simulink model "MATLAB_FILE_EV_final"  (R2021a)
settings: Solver=ode45  StartTime=0.0  StopTime=0.5  MaxStep=0.0001  RelTol=1e-3
undefined symbols (not defined in the file): Ion, Lithium
libraries: spsSeriesRLCBranchLib x14, spsIdealSwitchLib x10, pid_lib x9, spsMosfetLib x8, spsPWMGeneratorDCDCLib x6, spsVoltageMeasurementLib x5, spsThreePhaseSeriesRLCLoadLib x4, spsThreePhaseVIMeasurementLib x3, spsThreePhaseBreakerLib x2, spsUniversalBridgeLib x2, spsBatteryLib x1, spsThreePhaseSourceLib x1
(part 1 of 2)
settings Model: Creator=DarkDoom  LastModifiedBy=DarkDoom
settings SolverCC: ZeroCrossControl=DisableAll  SolverResetMethod=Robust

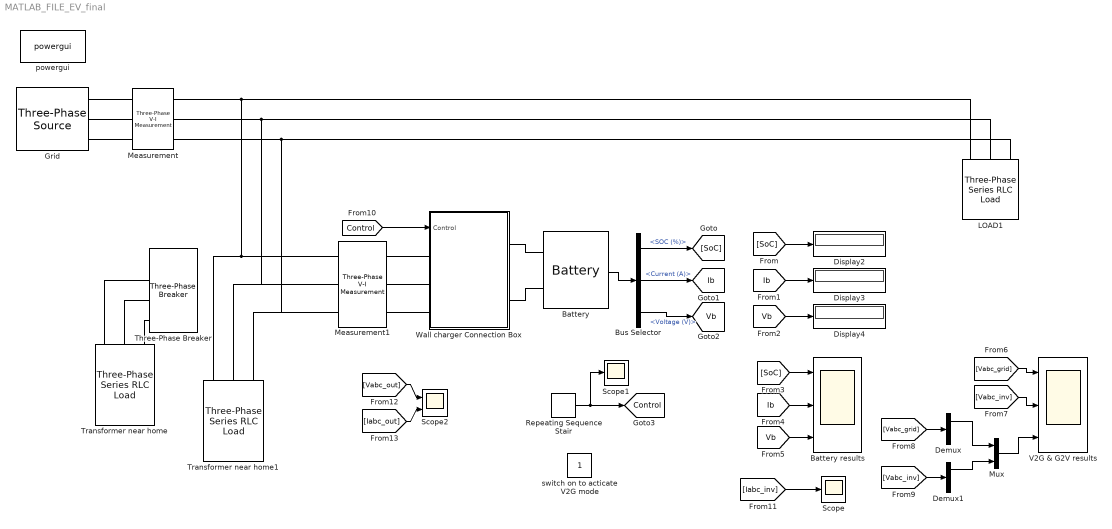
== system MATLAB_FILE_EV_final ==
  Battery : spsBatteryLib/Battery  BatType=Lithium-Ion  ShowTempParam=off  ThermalPreset=no  ShowAgeParam=off  NomV=230  NomQ=100  SOC=60  Batt_Tr=1e-3  PresetModel=on  MaxQ=100  MinV=172.5  FullV=267.717  Dis_rate=43.4783  R=0.023  Normal_OP=90.4348  expZone="[248.4887      4.913043]"  current=[6.5 13 32.5]  Units=Time  Tci=20  NomT=20  T2=-30  MaxQ2=4.8  FullV2=7.1  Normal_OP2=5.655  expZone2="[6.58           1]"  Rca=0.6  ti=2000  Dp=0  Neq0=0  Tsim=1e6  Ta1=25  Qeol=5.4*0.9  Reol=0.013333*1.2  Char_age=[2.3478, 3]  Dis_age=[2.3478, 10]  N1=1500  N2=10500  N3=1000  N4=1400  Ta2=45  N5=950
  Battery results : Scope  NumInputPorts=3
  Bus Selector : BusSelector  OutputSignals=SOC (%),Current (A),Voltage (V)
  Demux : Demux  Outputs=3
  Demux1 : Demux  Outputs=3
  Display2 : Display
  Display3 : Display
  Display4 : Display
  Grid : spsThreePhaseSourceLib/Three-Phase Source  InternalConnection=Yg  VoltagePhases=off  Voltage=380  PhaseAngle=0  Voltage_phases=[25e3 25e3 25e3]/sqrt(3)  PhaseAngles_phases=[0 -120 +120]  Frequency=50  NonIdealSource=on  SpecifyImpedance=on  Resistance=0.8929  Inductance=16.58e-3  ShortCircuitLevel=100e6  BaseVoltage=380  XRratio=7  BusType=swing  Pref=10e3  Qref=0  Prefabc=[10e3, 10e3, 10e3]  Qrefabc=[0, 0, 0]  Qmin=-inf  Qmax=inf
  LOAD1 : spsThreePhaseSeriesRLCLoadLib/Three-Phase Series RLC Load  LConnTagsString=A|B|C  Configuration=Y (grounded)  NominalVoltage=380  Vabc=[1e3 1e3 1e3]  Vabcp=[1e3 1e3 1e3]  NominalFrequency=50  UnbalancedPower=off  ActivePower=1e3  InductivePower=0  CapacitivePower=0  Pabc=[10e3 9e3 11e3]  QLabc=[100 90 110]  QCabc=[100 90 110]  Pabcp=[10e3 9e3 11e3]  QLabcp=[100 90 110]  QCabcp=[100 90 110]  Measurements=None  LoadType=constant Z
  Measurement : spsThreePhaseVIMeasurementLib/Three-Phase V-I Measurement  VoltageMeasurement=phase-to-ground  SetLabelV=on  LabelV=Vabc_grid  Vpu=off  VpuLL=off  CurrentMeasurement=yes  SetLabelI=on  LabelI=Iabc_grid  Ipu=off  Pbase=100e6  Vbase=500e3  OutputType=Complex  PhasorSimulation=off  PSBequivalent=0
  Measurement1 : spsThreePhaseVIMeasurementLib/Three-Phase V-I Measurement  VoltageMeasurement=phase-to-ground  SetLabelV=on  LabelV=Vabc_out  Vpu=off  VpuLL=off  CurrentMeasurement=yes  SetLabelI=on  LabelI=Iabc_out  Ipu=off  Pbase=100e6  Vbase=500e3  OutputType=Complex  PhasorSimulation=off  PSBequivalent=0
  Mux : Mux  Inputs=2
  Repeating Sequence Stair : simulink/Sources/Repeating Sequence Stair  OutValues=[0 0 1 1 0].'  tsamp=0.1  OutMin=[]  OutMax=[]  OutDataTypeStr=double  OutputDataTypeScalingMode=double  OutDataType=fixdt(0,8)  ConRadixGroup=Best Precision: Vector-wise  OutScaling=2^-12
  Scope : Scope
  Scope1 : Scope
  Scope2 : Scope  NumInputPorts=2
  Three-Phase Breaker : spsThreePhaseBreakerLib/Three-Phase Breaker  InitialState=open  SwitchA=on  SwitchB=on  SwitchC=on  SwitchTimes="[0.1  0.25]"  External=on  BreakerResistance=0.01  SnubberResistance=1e6  SnubberCapacitance=inf  Measurements=None
  Transformer near home : spsThreePhaseSeriesRLCLoadLib/Three-Phase Series RLC Load  LConnTagsString=A|B|C  Configuration=Y (grounded)  NominalVoltage=380  Vabc=[1e3 1e3 1e3]  Vabcp=[1e3 1e3 1e3]  NominalFrequency=50  UnbalancedPower=off  ActivePower=20e3  InductivePower=0  CapacitivePower=0  Pabc=[10e3 9e3 11e3]  QLabc=[100 90 110]  QCabc=[100 90 110]  Pabcp=[10e3 9e3 11e3]  QLabcp=[100 90 110]  QCabcp=[100 90 110]  Measurements=None  LoadType=constant Z
  Transformer near home1 : spsThreePhaseSeriesRLCLoadLib/Three-Phase Series RLC Load  LConnTagsString=A|B|C  Configuration=Y (grounded)  NominalVoltage=380  Vabc=[1e3 1e3 1e3]  Vabcp=[1e3 1e3 1e3]  NominalFrequency=50  UnbalancedPower=off  ActivePower=1e3  InductivePower=0  CapacitivePower=0  Pabc=[10e3 9e3 11e3]  QLabc=[100 90 110]  QCabc=[100 90 110]  Pabcp=[10e3 9e3 11e3]  QLabcp=[100 90 110]  QCabcp=[100 90 110]  Measurements=None  LoadType=constant Z
  V2G & G2V results : Scope  NumInputPorts=3
  Wall charger Connection Box : Subsystem
  powergui : spspowerguiLib/powergui  Priority=1  SimulationMode=Discrete  SampleTime=50e-6  frequency=60  Iterations=50  frequencyindice=0  Pbase=100e6  ErrMax=1e-4  UnitsV=kV  UnitsW=MW  buscounter=0  FunctionMessages=off  echomessages=off  EnableUseOfTLC=off  CurrentSourceSwitches=off  DisableSnubberDevices=off  DisableRonSwitches=off  DisableVfSwitches=off  DisplayEquations=off  AutomaticDiscreteSolvers=off  SolverType=Tustin/Backward Euler (TBE)  Interpol=off  ExternalGateDelay=off  methode=off  Ts=100  x0status=blocks  SPID=on  SwTol=0  HookPort=off  NonlinearTolerance=1e-4  nMaxIteration=100  ContinueOnMaxIteration=off  RestoreLinks=warning  ResistiveCurrentMeasurement=off  Frange=[0:2:500]  Ylog=off  Xlog=on  ShowGrid=off  save=off  variable=ZData  structure=0  ZoomFFT=off  StartTime=0.0  cycles=1  DisplayStyle=1  fundamental=60  FreqAxis=off  MaxFrequency=1000  frequencyindicesteady=1  RmsSteady=1  display=off
  switch on to acticate V2G mode : Constant  VectorParams1D=off
  tag scope: Control=global, Ib=global, Vb=global
  wires:
  [Control] -> Wall charger Connection Box/1(Control)
  Battery/1 -> Bus Selector/1
  Bus Selector/1 -> [SoC]  "<SOC (%)>"
  Bus Selector/2 -> [Ib]  "<Current (A)>"
  Bus Selector/3 -> [Vb]  "<Voltage (V)>"
  [SoC] -> Display2/1
  [Ib] -> Display3/1
  [Vb] -> Display4/1
  [SoC] -> Battery results/1
  [Ib] -> Battery results/2
  [Vb] -> Battery results/3
  [Vabc_grid] -> V2G & G2V results/1
  [Vabc_inv] -> V2G & G2V results/2
  [Vabc_grid] -> Demux/1
  [Vabc_inv] -> Demux1/1
  Demux/1 -> Mux/1
  Demux1/1 -> Mux/2
  Mux/1 -> V2G & G2V results/3
  [Iabc_inv] -> Scope/1
  Repeating Sequence Stair/1 -> [Control], Scope1/1
  [Vabc_out] -> Scope2/1
  [Iabc_out] -> Scope2/2
  connections:
  Grid/RConn1 -- Measurement/LConn1
  Grid/RConn2 -- Measurement/LConn2
  Grid/RConn3 -- Measurement/LConn3
  Transformer near home/LConn1 -- Three-Phase Breaker/LConn1
  Transformer near home/LConn2 -- Three-Phase Breaker/LConn2
  Transformer near home1/LConn3 -- Measurement1/LConn3 -- LOAD1/LConn3 -- Measurement/RConn3
  Wall charger Connection Box/RConn1 -- Battery/LConn1
  Wall charger Connection Box/RConn2 -- Battery/LConn2
  Wall charger Connection Box/LConn2 -- Measurement1/RConn2
  Wall charger Connection Box/LConn1 -- Measurement1/RConn1
  Wall charger Connection Box/LConn3 -- Measurement1/RConn3
  Transformer near home/LConn3 -- Three-Phase Breaker/LConn3
  Measurement1/LConn1 -- Transformer near home1/LConn1 -- Measurement/RConn1 -- LOAD1/LConn1
  Measurement/RConn2 -- Transformer near home1/LConn2 -- Measurement1/LConn2 -- LOAD1/LConn2

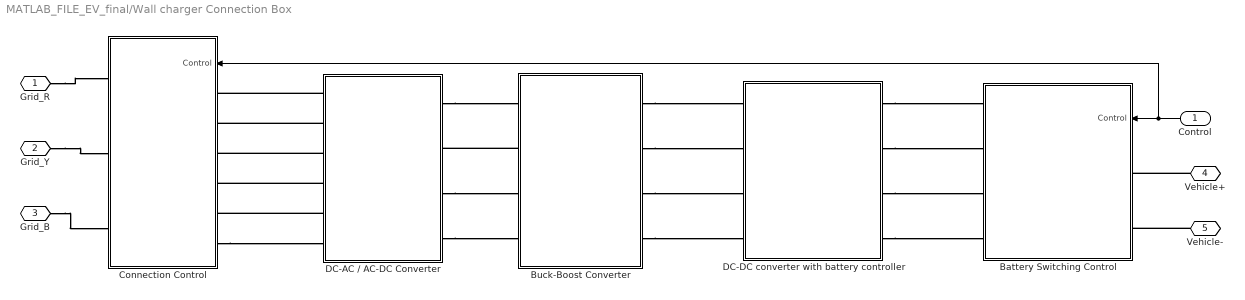
== system MATLAB_FILE_EV_final/Wall charger Connection Box ==
  Control : Inport
  Battery Switching Control : Subsystem
      settings: PortSchema="{\"entries\":[{\"content\":{\"sides\":[{\"content\":{\"connectorIds\":[\"LConn1\",\"LConn2\",\"LConn3\",\"LConn4\"]},\"type\":\"ConnectorPlacement.EquallySpacedRectSide\",\"uuid\":\"597ce45f-d2da-489f-9702-c83ae9b1152a\"},{\"content\":{\"connectorIds\":[\"In1\",\"RConn1\",\"RConn2\"],\"side\":\"RIGHT\"},\"type\":\"ConnectorPlacement.EquallySpacedRectSide\",\"uuid\":\"90ab1945-2787-45d6-b647-1c8eb49fe34d\"},{\"content\":{\"connectorIds\":[],\"side\":\"TOP\"},\"type\":\"ConnectorPlacement.EquallySpacedRectSide\",\"uuid\":\"5514c8fd-a1bb-4ed7-b1c0-08bce6a0e9e5\"}]},\"type\":\"ConnectorPlacement.EquallySpacedConnector\",\"uuid\":\"b6d566cb-31ba-40ab-ae9a-003997b713cb\"}],\"packageUris\":[\"http://schema.mathworks.com/mf0/Connector/R2020b\"],\"version\":\"1.0\"}"
  Buck-Boost Converter : Subsystem
  Connection Control : Subsystem
      settings: PortSchema="{\"entries\":[{\"content\":{\"sides\":[{\"content\":{\"connectorIds\":[\"LConn1\",\"LConn2\",\"LConn3\"]},\"type\":\"ConnectorPlacement.EquallySpacedRectSide\",\"uuid\":\"27ebf5cb-61b2-431e-8de2-c9344a0dfca5\"},{\"content\":{\"connectorIds\":[\"In1\",\"RConn1\",\"RConn2\",\"RConn3\",\"RConn4\",\"RConn5\",\"RConn6\"],\"side\":\"RIGHT\"},\"type\":\"ConnectorPlacement.EquallySpacedRectSide\",\"uuid\":\"2438100a-e43b-42f7-afa1-1af449516139\"},{\"content\":{\"connectorIds\":[],\"side\":\"TOP\"},\"type\":\"ConnectorPlacement.EquallySpacedRectSide\",\"uuid\":\"dcfa608d-f6dc-42e3-abf8-45a08af22825\"}]},\"type\":\"ConnectorPlacement.EquallySpacedConnector\",\"uuid\":\"5f0f36e8-f735-4489-a6f2-39fec655b509\"}],\"packageUris\":[\"http://schema.mathworks.com/mf0/Connector/R2020b\"],\"version\":\"1.0\"}"
  DC-AC / AC-DC Converter : Subsystem
  DC-DC converter with battery controller : Subsystem
  Grid_R : PMIOPort  Side=Left
  Grid_Y : PMIOPort  Port=2  Side=Left
  Grid_B : PMIOPort  Port=3  Side=Left
  Vehicle+ : PMIOPort  Port=4  Side=Right
  Vehicle- : PMIOPort  Port=5  Side=Right
  wires:
  Control/1 -> Connection Control/1(Control), Battery Switching Control/1(Control)
  connections:
  DC-AC / AC-DC Converter/LConn5 -- Connection Control/RConn5
  DC-AC / AC-DC Converter/LConn2 -- Connection Control/RConn2
  DC-DC converter with battery controller/RConn3 -- Battery Switching Control/LConn3
  Buck-Boost Converter/RConn2 -- DC-DC converter with battery controller/LConn2
  Grid_B/RConn1 -- Connection Control/LConn3
  DC-AC / AC-DC Converter/RConn3 -- Buck-Boost Converter/LConn3
  Grid_R/RConn1 -- Connection Control/LConn1
  DC-AC / AC-DC Converter/LConn1 -- Connection Control/RConn1
  Vehicle-/RConn1 -- Battery Switching Control/RConn2
  Vehicle+/RConn1 -- Battery Switching Control/RConn1
  Buck-Boost Converter/RConn4 -- DC-DC converter with battery controller/LConn4
  Grid_Y/RConn1 -- Connection Control/LConn2
  DC-AC / AC-DC Converter/LConn4 -- Connection Control/RConn4
  DC-DC converter with battery controller/RConn2 -- Battery Switching Control/LConn2
  DC-DC converter with battery controller/RConn1 -- Battery Switching Control/LConn1
  DC-DC converter with battery controller/RConn4 -- Battery Switching Control/LConn4
  Buck-Boost Converter/RConn1 -- DC-DC converter with battery controller/LConn1
  Buck-Boost Converter/LConn2 -- DC-AC / AC-DC Converter/RConn2
  DC-AC / AC-DC Converter/LConn3 -- Connection Control/RConn3
  DC-AC / AC-DC Converter/RConn1 -- Buck-Boost Converter/LConn1
  DC-AC / AC-DC Converter/RConn4 -- Buck-Boost Converter/LConn4
  Buck-Boost Converter/RConn3 -- DC-DC converter with battery controller/LConn3
  Connection Control/RConn6 -- DC-AC / AC-DC Converter/LConn6

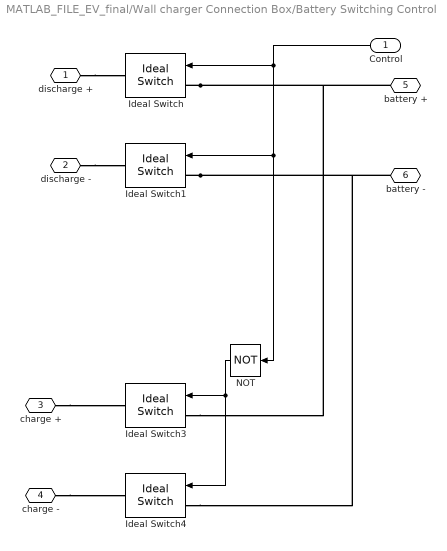
== system MATLAB_FILE_EV_final/Wall charger Connection Box/Battery Switching Control ==
  Control : Inport
  Ideal Switch{,1,3..4} (4 alike) : spsIdealSwitchLib/Ideal Switch  Ron=0.001  Lon=0  IC=0  Rs=1e5  Cs=inf  Measurements=off
  NOT : Logic  Operator=NOT  IconShape=distinctive  AllPortsSameDT=off  OutDataTypeStr=boolean
  discharge + : PMIOPort  Side=Left
  discharge - : PMIOPort  Port=2  Side=Left
  charge + : PMIOPort  Port=3  Side=Left
  charge - : PMIOPort  Port=4  Side=Left
  battery + : PMIOPort  Port=5  Side=Right
  battery - : PMIOPort  Port=6  Side=Right
  wires:
  Control/1 -> NOT/1, Ideal Switch1/1, Ideal Switch/1
  NOT/1 -> Ideal Switch4/1, Ideal Switch3/1
  connections:
  charge -/RConn1 -- Ideal Switch4/RConn1
  discharge +/RConn1 -- Ideal Switch/RConn1
  Ideal Switch1/LConn1 -- battery -/RConn1 -- Ideal Switch4/LConn1
  discharge -/RConn1 -- Ideal Switch1/RConn1
  Ideal Switch/LConn1 -- battery +/RConn1 -- Ideal Switch3/LConn1
  charge +/RConn1 -- Ideal Switch3/RConn1

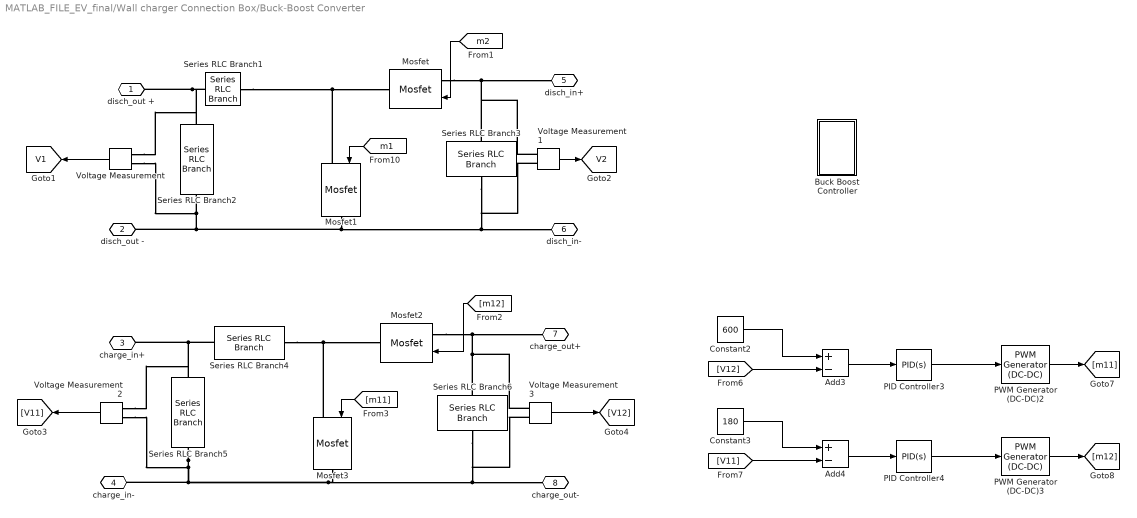
== system MATLAB_FILE_EV_final/Wall charger Connection Box/Buck-Boost Converter ==
  Add3 : Sum  Inputs=+-
  Add4 : Sum  Inputs=+-
  Buck Boost Controller : Subsystem
  Constant2 : Constant  Value=600
  Constant3 : Constant  Value=180
  Mosfet{,1..3} (4 alike) : spsMosfetLib/Mosfet  Ron=0.1  Lon=0  Rd=0.01  Vfd=0  IC=0  Rs=1e5  Cs=inf  Measurements=off
  PID Controller3 : pid_lib/PID Controller  Controller=PID  Form=Parallel  TimeDomain=Continuous-time  UseExternalTs=off  SampleTime=-1  IntegratorMethod=Forward Euler  FilterMethod=Forward Euler  ControllerParametersSource=internal  P=0  I=7  D=0  UseFilter=on  N=100  TunerSelectOption=Transfer Function Based (PID Tuner App)  InitialConditionSource=internal  InitialConditionForIntegrator=0  InitialConditionForFilter=0  DifferentiatorICPrevScaledInput=0  ExternalReset=none  TrackingMode=off  Kt=1  LimitOutput=off  SatLimitsSource=internal  UpperSaturationLimit=inf  LowerSaturationLimit=-inf  LinearizeAsGain=on  AntiWindupMode=none  Kb=1  POutMin=[]  POutMax=[]  IOutMin=[]  IOutMax=[]  DOutMin=[]  DOutMax=[]  NOutMin=[]  NOutMax=[]  SumOutMin=[]  SumOutMax=[]  SaturationOutMin=[]  SaturationOutMax=[]  PParamMin=[]  PParamMax=[]  IParamMin=[]  IParamMax=[]  DParamMin=[]  DParamMax=[]  NParamMin=[]  NParamMax=[]  KbParamMin=[]  KbParamMax=[]  KtParamMin=[]  KtParamMax=[]  KbOutMin=[]  KbOutMax=[]  KtOutMin=[]  KtOutMax=[]  IntegratorOutMin=[]  IntegratorOutMax=[]  FilterOutMin=[]  FilterOutMax=[]  SumI1OutMin=[]  SumI1OutMax=[]  SumI2OutMin=[]  SumI2OutMax=[]  SumI3OutMin=[]  SumI3OutMax=[]  SumI4OutMin=[]  SumI4OutMax=[]  SumDOutMin=[]  SumDOutMax=[]  DifferentiatorOutMin=[]  DifferentiatorOutMax=[]  FilterDiffOutCoefMin=[]  FilterDiffOutCoefMax=[]  ReciprocalOutMin=[]  ReciprocalOutMax=[]  SumDenOutMin=[]  SumDenOutMax=[]  SumNumOutMin=[]  SumNumOutMax=[]  DivideOutMin=[]  DivideOutMax=[]  UdiffTsProdOutMin=[]  UdiffTsProdOutMax=[]  NTsProdOutMin=[]  NTsProdOutMax=[]  UintegralTsProdOutMin=[]  UintegralTsProdOutMax=[]  UngainTsProdOutMin=[]  UngainTsProdOutMax=[]  IntegratorContinuousStateAttributes=''  IntegratorStateMustResolveToSignalObject=off  IntegratorRTWStateStorageClass=Auto  FilterContinuousStateAttributes=''  FilterStateMustResolveToSignalObject=off  FilterRTWStateStorageClass=Auto  ParallelPVariant=InternalParameters  IdealPVariant=Disabled  IVariant=InternalParameters  DVariant=InternalParameters  IntegratorVariant=Continuous  SatVariant=Disabled  AWVariant=Passthrough  PCopyVariant=Disabled  TRVariant=Disabled  FdbkBlocksVariant=Forward  IdealPFdbkVariant=Disabled  SatFdbkVariant=Disabled  DerivativeFilterVariant=ContFilter  NVariant=InternalParameters  NCopyVariant=Disabled  FilterICVariant=InternalICsFilter  IntegratorICVariant=InternalICs  ExternalResetVariant=Disabled  TRSumVariant=Passthrough  SumFdbkVariant=Disabled  SumVariant=Sum_PID  TsampFilterVariant=InternalTs  TsampNgainVariant=Passthrough  TsampIntegralVariant=Passthrough  ExternalSaturationOutDataTypeStr=Inherit: Same as second input
  PID Controller4 : pid_lib/PID Controller  Controller=PID  Form=Parallel  TimeDomain=Continuous-time  UseExternalTs=off  SampleTime=-1  IntegratorMethod=Forward Euler  FilterMethod=Forward Euler  ControllerParametersSource=internal  P=0  I=7  D=0  UseFilter=on  N=100  TunerSelectOption=Transfer Function Based (PID Tuner App)  InitialConditionSource=internal  InitialConditionForIntegrator=0  InitialConditionForFilter=0  DifferentiatorICPrevScaledInput=0  ExternalReset=none  TrackingMode=off  Kt=1  LimitOutput=off  SatLimitsSource=internal  UpperSaturationLimit=inf  LowerSaturationLimit=-inf  LinearizeAsGain=on  AntiWindupMode=none  Kb=1  POutMin=[]  POutMax=[]  IOutMin=[]  IOutMax=[]  DOutMin=[]  DOutMax=[]  NOutMin=[]  NOutMax=[]  SumOutMin=[]  SumOutMax=[]  SaturationOutMin=[]  SaturationOutMax=[]  PParamMin=[]  PParamMax=[]  IParamMin=[]  IParamMax=[]  DParamMin=[]  DParamMax=[]  NParamMin=[]  NParamMax=[]  KbParamMin=[]  KbParamMax=[]  KtParamMin=[]  KtParamMax=[]  KbOutMin=[]  KbOutMax=[]  KtOutMin=[]  KtOutMax=[]  IntegratorOutMin=[]  IntegratorOutMax=[]  FilterOutMin=[]  FilterOutMax=[]  SumI1OutMin=[]  SumI1OutMax=[]  SumI2OutMin=[]  SumI2OutMax=[]  SumI3OutMin=[]  SumI3OutMax=[]  SumI4OutMin=[]  SumI4OutMax=[]  SumDOutMin=[]  SumDOutMax=[]  DifferentiatorOutMin=[]  DifferentiatorOutMax=[]  FilterDiffOutCoefMin=[]  FilterDiffOutCoefMax=[]  ReciprocalOutMin=[]  ReciprocalOutMax=[]  SumDenOutMin=[]  SumDenOutMax=[]  SumNumOutMin=[]  SumNumOutMax=[]  DivideOutMin=[]  DivideOutMax=[]  UdiffTsProdOutMin=[]  UdiffTsProdOutMax=[]  NTsProdOutMin=[]  NTsProdOutMax=[]  UintegralTsProdOutMin=[]  UintegralTsProdOutMax=[]  UngainTsProdOutMin=[]  UngainTsProdOutMax=[]  IntegratorContinuousStateAttributes=''  IntegratorStateMustResolveToSignalObject=off  IntegratorRTWStateStorageClass=Auto  FilterContinuousStateAttributes=''  FilterStateMustResolveToSignalObject=off  FilterRTWStateStorageClass=Auto  ParallelPVariant=InternalParameters  IdealPVariant=Disabled  IVariant=InternalParameters  DVariant=InternalParameters  IntegratorVariant=Continuous  SatVariant=Disabled  AWVariant=Passthrough  PCopyVariant=Disabled  TRVariant=Disabled  FdbkBlocksVariant=Forward  IdealPFdbkVariant=Disabled  SatFdbkVariant=Disabled  DerivativeFilterVariant=ContFilter  NVariant=InternalParameters  NCopyVariant=Disabled  FilterICVariant=InternalICsFilter  IntegratorICVariant=InternalICs  ExternalResetVariant=Disabled  TRSumVariant=Passthrough  SumFdbkVariant=Disabled  SumVariant=Sum_PID  TsampFilterVariant=InternalTs  TsampNgainVariant=Passthrough  TsampIntegralVariant=Passthrough  ExternalSaturationOutDataTypeStr=Inherit: Same as second input
  PWM Generator (DC-DC)2 : spsPWMGeneratorDCDCLib/PWM Generator (DC-DC)  Fsw=5000  Ts=0
  PWM Generator (DC-DC)3 : spsPWMGeneratorDCDCLib/PWM Generator (DC-DC)  Fsw=5000  Ts=0
  Series RLC Branch1 : spsSeriesRLCBranchLib/Series RLC Branch  LConnTagsString=__new0  RConnTagsString=__new0  BranchType=L  Resistance=1  Inductance=1e-3  SetiL0=off  InitialCurrent=0  Capacitance=1e-6  Setx0=off  InitialVoltage=0  Measurements=None
  Series RLC Branch{2..3,5..6} (4 alike) : spsSeriesRLCBranchLib/Series RLC Branch  LConnTagsString=__new0  RConnTagsString=__new0  BranchType=RC  Resistance=0.0001  Inductance=1e-3  SetiL0=off  InitialCurrent=0  Capacitance=1000e-6  Setx0=off  InitialVoltage=0  Measurements=None
  Series RLC Branch4 : spsSeriesRLCBranchLib/Series RLC Branch  LConnTagsString=__new0  RConnTagsString=__new0  BranchType=L  Resistance=100e3  Inductance=1e-3  SetiL0=off  InitialCurrent=0  Capacitance=1e-6  Setx0=off  InitialVoltage=0  Measurements=None
  Voltage Measurement{,1..3} (4 alike) : spsVoltageMeasurementLib/Voltage Measurement  PhasorSimulation=off  OutputType=Complex  PSBequivalent=0
  disch_out + : PMIOPort  Side=Left
  disch_out - : PMIOPort  Port=2  Side=Left
  charge_in+ : PMIOPort  Port=3  Side=Left
  charge_in- : PMIOPort  Port=4  Side=Left
  disch_in+ : PMIOPort  Port=5  Side=Right
  disch_in- : PMIOPort  Port=6  Side=Right
  charge_out+ : PMIOPort  Port=7  Side=Right
  charge_out- : PMIOPort  Port=8  Side=Right
  tag scope: V1=global, V2=global
  wires:
  Voltage Measurement1/1 -> [V2]
  Voltage Measurement/1 -> [V1]
  PWM Generator (DC-DC)2/1 -> [m11]
  [V11] -> Add4/2
  Add3/1 -> PID Controller3/1
  Voltage Measurement3/1 -> [V12]
  PID Controller4/1 -> PWM Generator (DC-DC)3/1
  PID Controller3/1 -> PWM Generator (DC-DC)2/1
  Add4/1 -> PID Controller4/1
  [m11] -> Mosfet3/1
  Voltage Measurement2/1 -> [V11]
  PWM Generator (DC-DC)3/1 -> [m12]
  [m12] -> Mosfet2/1
  Constant3/1 -> Add4/1
  Constant2/1 -> Add3/1
  [V12] -> Add3/2
  [m1] -> Mosfet1/1
  [m2] -> Mosfet/1
  connections:
  Series RLC Branch5/RConn1 -- charge_in-/RConn1 -- charge_out-/RConn1 -- Voltage Measurement3/LConn2 -- Series RLC Branch6/RConn1 -- Mosfet3/RConn1 -- Voltage Measurement2/LConn2
  Mosfet1/RConn1 -- disch_in-/RConn1 -- Voltage Measurement1/LConn2 -- Series RLC Branch3/RConn1 -- disch_out -/RConn1 -- Voltage Measurement/LConn2 -- Series RLC Branch2/RConn1
  Mosfet/LConn1 -- disch_in+/RConn1 -- Voltage Measurement1/LConn1 -- Series RLC Branch3/LConn1
  Series RLC Branch4/LConn1 -- charge_in+/RConn1 -- Voltage Measurement2/LConn1 -- Series RLC Branch5/LConn1
  Series RLC Branch1/LConn1 -- Voltage Measurement/LConn1 -- Series RLC Branch2/LConn1 -- disch_out +/RConn1
  Series RLC Branch6/LConn1 -- Voltage Measurement3/LConn1 -- charge_out+/RConn1 -- Mosfet2/LConn1
  Mosfet1/LConn1 -- Series RLC Branch1/RConn1 -- Mosfet/RConn1
  Series RLC Branch4/RConn1 -- Mosfet3/LConn1 -- Mosfet2/RConn1

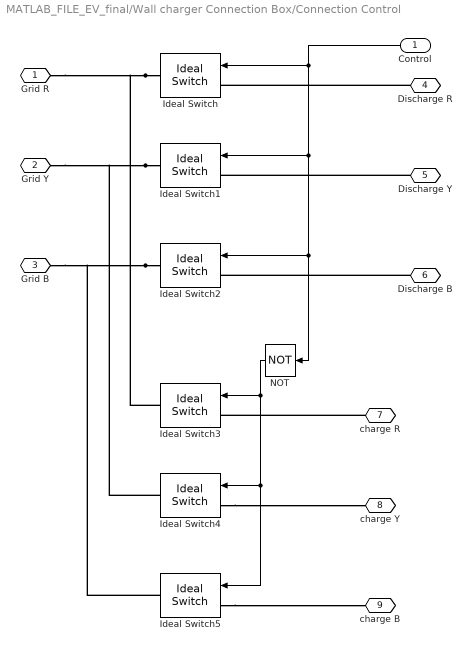
== system MATLAB_FILE_EV_final/Wall charger Connection Box/Connection Control ==
  Control : Inport
  Ideal Switch{,1..5} (6 alike) : spsIdealSwitchLib/Ideal Switch  Ron=0.001  Lon=0  IC=0  Rs=1e5  Cs=inf  Measurements=off
  NOT : Logic  Operator=NOT  IconShape=distinctive  AllPortsSameDT=off  OutDataTypeStr=boolean
  Grid R : PMIOPort  Side=Left
  Grid Y : PMIOPort  Port=2  Side=Left
  Grid B : PMIOPort  Port=3  Side=Left
  Discharge R : PMIOPort  Port=4  Side=Right
  Discharge Y : PMIOPort  Port=5  Side=Right
  Discharge B : PMIOPort  Port=6  Side=Right
  charge R : PMIOPort  Port=7  Side=Right
  charge Y : PMIOPort  Port=8  Side=Right
  charge B : PMIOPort  Port=9  Side=Right
  wires:
  Control/1 -> NOT/1, Ideal Switch2/1, Ideal Switch1/1, Ideal Switch/1
  NOT/1 -> Ideal Switch5/1, Ideal Switch4/1, Ideal Switch3/1
  connections:
  Ideal Switch2/RConn1 -- Grid B/RConn1 -- Ideal Switch5/RConn1
  Discharge R/RConn1 -- Ideal Switch/LConn1
  Discharge B/RConn1 -- Ideal Switch2/LConn1
  Ideal Switch/RConn1 -- Grid R/RConn1 -- Ideal Switch3/RConn1
  Ideal Switch1/RConn1 -- Grid Y/RConn1 -- Ideal Switch4/RConn1
  Ideal Switch4/LConn1 -- charge Y/RConn1
  Discharge Y/RConn1 -- Ideal Switch1/LConn1
  charge R/RConn1 -- Ideal Switch3/LConn1
  Ideal Switch5/LConn1 -- charge B/RConn1

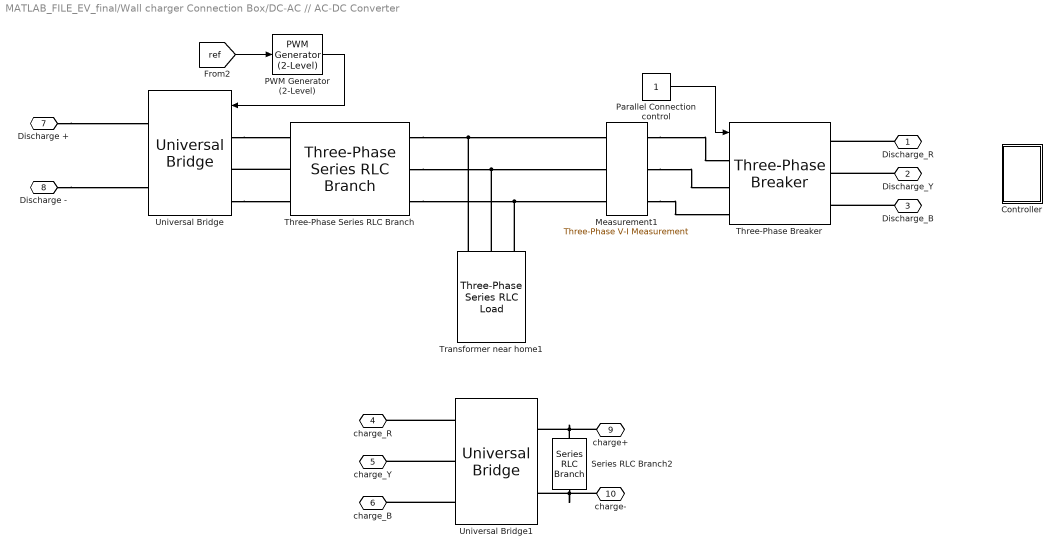
== system MATLAB_FILE_EV_final/Wall charger Connection Box/DC-AC // AC-DC Converter ==
  Controller : Subsystem
  Measurement1 : spsThreePhaseVIMeasurementLib/Three-Phase V-I Measurement  VoltageMeasurement=phase-to-ground  SetLabelV=on  LabelV=Vabc_inv  Vpu=off  VpuLL=off  CurrentMeasurement=yes  SetLabelI=on  LabelI=Iabc_inv  Ipu=off  Pbase=100e6  Vbase=500e3  OutputType=Complex  PhasorSimulation=off  PSBequivalent=0
  PWM Generator (2-Level) : spsPWMGenerator2LevelLib/PWM Generator (2-Level)  ModulatorType=Three-phase bridge (6 pulses)  ModulatorMode=Unsynchronized  Fc=4950  Pc=90  nF=27  MinMax="[ -1  1 ]"  SamplingTechnique=Natural  ModulatingSignals=off  m=0.8  Freq=60  Phase=0  Ts=2.02e-6  ShowCarrierOutport=off
  Parallel Connection control : Constant
  Series RLC Branch2 : spsSeriesRLCBranchLib/Series RLC Branch  LConnTagsString=__new0  RConnTagsString=__new0  BranchType=RC  Resistance=10e3  Inductance=1e-3  SetiL0=off  InitialCurrent=0  Capacitance=1000e-6  Setx0=off  InitialVoltage=0  Measurements=None
  Three-Phase Series RLC Branch : spsThreePhaseSeriesRLCBranchLib/Three-Phase Series RLC Branch  LConnTagsString=A|B|C  RConnTagsString=A|B|C  BranchType=RL  Resistance=0.004332  Inductance=0.0013789184  Capacitance=1e-6  Measurements=None
  Three-Phase Breaker : spsThreePhaseBreakerLib/Three-Phase Breaker  InitialState=open  SwitchA=on  SwitchB=on  SwitchC=on  SwitchTimes="[1/60  5/60]"  External=on  BreakerResistance=0.01  SnubberResistance=1e6  SnubberCapacitance=inf  Measurements=None
  Transformer near home1 : spsThreePhaseSeriesRLCLoadLib/Three-Phase Series RLC Load  LConnTagsString=A|B|C  Configuration=Delta  NominalVoltage=380  Vabc=[1e3 1e3 1e3]  Vabcp=[1e3 1e3 1e3]  NominalFrequency=50  UnbalancedPower=off  ActivePower=100  InductivePower=0  CapacitivePower=5000  Pabc=[10e3 9e3 11e3]  QLabc=[100 90 110]  QCabc=[100 90 110]  Pabcp=[10e3 9e3 11e3]  QLabcp=[100 90 110]  QCabcp=[100 90 110]  Measurements=None  LoadType=constant Z
  Universal Bridge : spsUniversalBridgeLib/Universal Bridge  Arms=3  SnubberResistance=1e5  SnubberCapacitance=inf  Device=IGBT / Diodes  Ron=1e-3  Lon=0  ForwardVoltages="[  0  0  ]"  ForwardVoltage=0  GTOparameters=[ 10e-6 , 20e-6 ]  IGBTparameters=[ 1e-6 , 2e-6 ]  Measurements=None  Measurements_2=None  converterType=Rectifier
  Universal Bridge1 : spsUniversalBridgeLib/Universal Bridge  Arms=3  SnubberResistance=1e5  SnubberCapacitance=inf  Device=Diodes  Ron=1e-3  Lon=0  ForwardVoltages="[  0  0  ]"  ForwardVoltage=0  GTOparameters=[ 10e-6 , 20e-6 ]  IGBTparameters=[ 1e-6 , 2e-6 ]  Measurements=None  Measurements_2=None  converterType=Rectifier
  Discharge_R : PMIOPort  Side=Left
  Discharge_Y : PMIOPort  Port=2  Side=Left
  Discharge_B : PMIOPort  Port=3  Side=Left
  charge_R : PMIOPort  Port=4  Side=Left
  charge_Y : PMIOPort  Port=5  Side=Left
  charge_B : PMIOPort  Port=6  Side=Left
  Discharge + : PMIOPort  Port=7  Side=Right
  Discharge - : PMIOPort  Port=8  Side=Right
  charge+ : PMIOPort  Port=9  Side=Right
  charge- : PMIOPort  Port=10  Side=Right
  wires:
  PWM Generator (2-Level)/1 -> Universal Bridge/1
  Parallel Connection control/1 -> Three-Phase Breaker/1
  [ref] -> PWM Generator (2-Level)/1
  connections:
  Universal Bridge1/LConn2 -- charge_Y/RConn1
  Universal Bridge1/LConn3 -- charge_B/RConn1
  Discharge_Y/RConn1 -- Three-Phase Breaker/RConn2
  Three-Phase Series RLC Branch/RConn1 -- Transformer near home1/LConn1 -- Measurement1/LConn1
  Measurement1/RConn2 -- Three-Phase Breaker/LConn2
  charge-/RConn1 -- Series RLC Branch2/RConn1 -- Universal Bridge1/RConn2
  Three-Phase Series RLC Branch/RConn3 -- Measurement1/LConn3 -- Transformer near home1/LConn3
  Discharge_B/RConn1 -- Three-Phase Breaker/RConn3
  Three-Phase Series RLC Branch/LConn2 -- Universal Bridge/LConn2
  Universal Bridge/LConn1 -- Three-Phase Series RLC Branch/LConn1
  Discharge -/RConn1 -- Universal Bridge/RConn2
  Universal Bridge/LConn3 -- Three-Phase Series RLC Branch/LConn3
  Three-Phase Series RLC Branch/RConn2 -- Measurement1/LConn2 -- Transformer near home1/LConn2
  Discharge +/RConn1 -- Universal Bridge/RConn1
  charge+/RConn1 -- Series RLC Branch2/LConn1 -- Universal Bridge1/RConn1
  Discharge_R/RConn1 -- Three-Phase Breaker/RConn1
  Measurement1/RConn1 -- Three-Phase Breaker/LConn1
  Measurement1/RConn3 -- Three-Phase Breaker/LConn3
  Universal Bridge1/LConn1 -- charge_R/RConn1

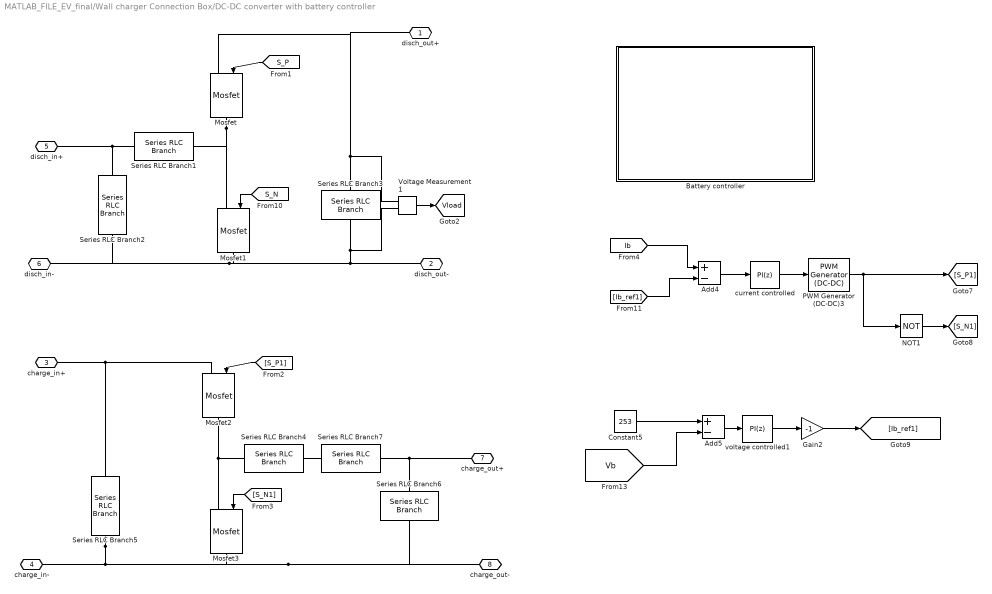
== system MATLAB_FILE_EV_final/Wall charger Connection Box/DC-DC converter with battery controller ==
  Add4 : Sum  Inputs=+-
  Add5 : Sum  Inputs=+-
  Battery controller : Subsystem
  Constant5 : Constant  Value=253
  Gain2 : Gain  Gain=-1
  Mosfet{,1..3} (4 alike) : spsMosfetLib/Mosfet  Ron=0.1  Lon=0  Rd=0.01  Vfd=0  IC=0  Rs=1e5  Cs=inf  Measurements=off
  NOT1 : Logic  Operator=NOT  IconShape=distinctive  AllPortsSameDT=off  OutDataTypeStr=boolean
  PWM Generator (DC-DC)3 : spsPWMGeneratorDCDCLib/PWM Generator (DC-DC)  Fsw=10e3  Ts=5e-6
  Series RLC Branch1 : spsSeriesRLCBranchLib/Series RLC Branch  LConnTagsString=__new0  RConnTagsString=__new0  BranchType=RL  Resistance=1000  Inductance=5.76e-4  SetiL0=off  InitialCurrent=0  Capacitance=1e-6  Setx0=off  InitialVoltage=0  Measurements=None
  Series RLC Branch2 : spsSeriesRLCBranchLib/Series RLC Branch  LConnTagsString=__new0  RConnTagsString=__new0  BranchType=R  Resistance=10  Inductance=1e-3  SetiL0=off  InitialCurrent=0  Capacitance=1000e-6  Setx0=off  InitialVoltage=0  Measurements=None
  Series RLC Branch3 : spsSeriesRLCBranchLib/Series RLC Branch  LConnTagsString=__new0  RConnTagsString=__new0  BranchType=RC  Resistance=0.001  Inductance=1e-3  SetiL0=off  InitialCurrent=0  Capacitance=1000e-6  Setx0=off  InitialVoltage=0  Measurements=None
  Series RLC Branch4 : spsSeriesRLCBranchLib/Series RLC Branch  LConnTagsString=__new0  RConnTagsString=__new0  BranchType=RL  Resistance=0.05  Inductance=5.76e-4  SetiL0=off  InitialCurrent=0  Capacitance=1000e-6  Setx0=off  InitialVoltage=0  Measurements=None
  Series RLC Branch5 : spsSeriesRLCBranchLib/Series RLC Branch  LConnTagsString=__new0  RConnTagsString=__new0  BranchType=RC  Resistance=0.001  Inductance=1e-3  SetiL0=off  InitialCurrent=0  Capacitance=1000e-6  Setx0=off  InitialVoltage=0  Measurements=None
  Series RLC Branch6 : spsSeriesRLCBranchLib/Series RLC Branch  LConnTagsString=__new0  RConnTagsString=__new0  BranchType=RC  Resistance=1e-3  Inductance=1e-3  SetiL0=off  InitialCurrent=0  Capacitance=5600e-6  Setx0=off  InitialVoltage=0  Measurements=None
  Series RLC Branch7 : spsSeriesRLCBranchLib/Series RLC Branch  LConnTagsString=__new0  RConnTagsString=__new0  BranchType=R  Resistance=10  Inductance=1e-3  SetiL0=off  InitialCurrent=0  Capacitance=1000e-6  Setx0=off  InitialVoltage=0  Measurements=None
  Voltage Measurement1 : spsVoltageMeasurementLib/Voltage Measurement  PhasorSimulation=off  OutputType=Complex  PSBequivalent=0
  current controlled : pid_lib/PID Controller  Controller=PI  Form=Parallel  TimeDomain=Discrete-time  UseExternalTs=off  SampleTime=500e-6  IntegratorMethod=Forward Euler  FilterMethod=Forward Euler  ControllerParametersSource=internal  P=0.005  I=10  D=0  UseFilter=on  N=100  TunerSelectOption=Transfer Function Based (PID Tuner App)  InitialConditionSource=internal  InitialConditionForIntegrator=0.54  InitialConditionForFilter=0  DifferentiatorICPrevScaledInput=0  ExternalReset=none  TrackingMode=off  Kt=1  LimitOutput=on  SatLimitsSource=internal  UpperSaturationLimit=0.95  LowerSaturationLimit=0  LinearizeAsGain=on  AntiWindupMode=none  Kb=1  POutMin=[]  POutMax=[]  IOutMin=[]  IOutMax=[]  DOutMin=[]  DOutMax=[]  NOutMin=[]  NOutMax=[]  SumOutMin=[]  SumOutMax=[]  SaturationOutMin=[]  SaturationOutMax=[]  PParamMin=[]  PParamMax=[]  IParamMin=[]  IParamMax=[]  DParamMin=[]  DParamMax=[]  NParamMin=[]  NParamMax=[]  KbParamMin=[]  KbParamMax=[]  KtParamMin=[]  KtParamMax=[]  KbOutMin=[]  KbOutMax=[]  KtOutMin=[]  KtOutMax=[]  IntegratorOutMin=[]  IntegratorOutMax=[]  FilterOutMin=[]  FilterOutMax=[]  SumI1OutMin=[]  SumI1OutMax=[]  SumI2OutMin=[]  SumI2OutMax=[]  SumI3OutMin=[]  SumI3OutMax=[]  SumI4OutMin=[]  SumI4OutMax=[]  SumDOutMin=[]  SumDOutMax=[]  DifferentiatorOutMin=[]  DifferentiatorOutMax=[]  FilterDiffOutCoefMin=[]  FilterDiffOutCoefMax=[]  ReciprocalOutMin=[]  ReciprocalOutMax=[]  SumDenOutMin=[]  SumDenOutMax=[]  SumNumOutMin=[]  SumNumOutMax=[]  DivideOutMin=[]  DivideOutMax=[]  UdiffTsProdOutMin=[]  UdiffTsProdOutMax=[]  NTsProdOutMin=[]  NTsProdOutMax=[]  UintegralTsProdOutMin=[]  UintegralTsProdOutMax=[]  UngainTsProdOutMin=[]  UngainTsProdOutMax=[]  IntegratorContinuousStateAttributes=''  IntegratorStateMustResolveToSignalObject=off  IntegratorRTWStateStorageClass=Auto  FilterContinuousStateAttributes=''  FilterStateMustResolveToSignalObject=off  FilterRTWStateStorageClass=Auto  ParallelPVariant=InternalParameters  IdealPVariant=Disabled  IVariant=InternalParameters  DVariant=Disabled  IntegratorVariant=Discrete  SatVariant=Enabled  AWVariant=Passthrough  PCopyVariant=Disabled  TRVariant=Disabled  FdbkBlocksVariant=Forward  IdealPFdbkVariant=Disabled  SatFdbkVariant=Disabled  DerivativeFilterVariant=Disabled  NVariant=Disabled  NCopyVariant=Disabled_SignalSpec  FilterICVariant=Disabled  IntegratorICVariant=InternalICs  ExternalResetVariant=Disabled  TRSumVariant=Passthrough  SumFdbkVariant=Disabled  SumVariant=Sum_PI  TsampFilterVariant=InternalTs  TsampNgainVariant=Passthrough  TsampIntegralVariant=Passthrough  ExternalSaturationOutDataTypeStr=Inherit: Same as second input
  voltage controlled1 : pid_lib/PID Controller  Controller=PI  Form=Parallel  TimeDomain=Discrete-time  UseExternalTs=off  SampleTime=500e-6  IntegratorMethod=Forward Euler  FilterMethod=Forward Euler  ControllerParametersSource=internal  P=40  I=2000  D=0  UseFilter=on  N=100  TunerSelectOption=Transfer Function Based (PID Tuner App)  InitialConditionSource=internal  InitialConditionForIntegrator=0  InitialConditionForFilter=0  DifferentiatorICPrevScaledInput=0  ExternalReset=none  TrackingMode=off  Kt=1  LimitOutput=on  SatLimitsSource=internal  UpperSaturationLimit=22  LowerSaturationLimit=0  LinearizeAsGain=on  AntiWindupMode=none  Kb=1  POutMin=[]  POutMax=[]  IOutMin=[]  IOutMax=[]  DOutMin=[]  DOutMax=[]  NOutMin=[]  NOutMax=[]  SumOutMin=[]  SumOutMax=[]  SaturationOutMin=[]  SaturationOutMax=[]  PParamMin=[]  PParamMax=[]  IParamMin=[]  IParamMax=[]  DParamMin=[]  DParamMax=[]  NParamMin=[]  NParamMax=[]  KbParamMin=[]  KbParamMax=[]  KtParamMin=[]  KtParamMax=[]  KbOutMin=[]  KbOutMax=[]  KtOutMin=[]  KtOutMax=[]  IntegratorOutMin=[]  IntegratorOutMax=[]  FilterOutMin=[]  FilterOutMax=[]  SumI1OutMin=[]  SumI1OutMax=[]  SumI2OutMin=[]  SumI2OutMax=[]  SumI3OutMin=[]  SumI3OutMax=[]  SumI4OutMin=[]  SumI4OutMax=[]  SumDOutMin=[]  SumDOutMax=[]  DifferentiatorOutMin=[]  DifferentiatorOutMax=[]  FilterDiffOutCoefMin=[]  FilterDiffOutCoefMax=[]  ReciprocalOutMin=[]  ReciprocalOutMax=[]  SumDenOutMin=[]  SumDenOutMax=[]  SumNumOutMin=[]  SumNumOutMax=[]  DivideOutMin=[]  DivideOutMax=[]  UdiffTsProdOutMin=[]  UdiffTsProdOutMax=[]  NTsProdOutMin=[]  NTsProdOutMax=[]  UintegralTsProdOutMin=[]  UintegralTsProdOutMax=[]  UngainTsProdOutMin=[]  UngainTsProdOutMax=[]  IntegratorContinuousStateAttributes=''  IntegratorStateMustResolveToSignalObject=off  IntegratorRTWStateStorageClass=Auto  FilterContinuousStateAttributes=''  FilterStateMustResolveToSignalObject=off  FilterRTWStateStorageClass=Auto  ParallelPVariant=InternalParameters  IdealPVariant=Disabled  IVariant=InternalParameters  DVariant=Disabled  IntegratorVariant=Discrete  SatVariant=Enabled  AWVariant=Passthrough  PCopyVariant=Disabled  TRVariant=Disabled  FdbkBlocksVariant=Forward  IdealPFdbkVariant=Disabled  SatFdbkVariant=Disabled  DerivativeFilterVariant=Disabled  NVariant=Disabled  NCopyVariant=Disabled_SignalSpec  FilterICVariant=Disabled  IntegratorICVariant=InternalICs  ExternalResetVariant=Disabled  TRSumVariant=Passthrough  SumFdbkVariant=Disabled  SumVariant=Sum_PI  TsampFilterVariant=InternalTs  TsampNgainVariant=Passthrough  TsampIntegralVariant=Passthrough  ExternalSaturationOutDataTypeStr=Inherit: Same as second input
  disch_out+ : PMIOPort  Side=Left
  disch_out- : PMIOPort  Port=2  Side=Left
  charge_in+ : PMIOPort  Port=3  Side=Left
  charge_in- : PMIOPort  Port=4  Side=Left
  disch_in+ : PMIOPort  Port=5  Side=Right
  disch_in- : PMIOPort  Port=6  Side=Right
  charge_out+ : PMIOPort  Port=7  Side=Right
  charge_out- : PMIOPort  Port=8  Side=Right
  tag scope: Vload=global
  wires:
  [S_P1] -> Mosfet2/1
  Add5/1 -> voltage controlled1/1
  [S_N1] -> Mosfet3/1
  PWM Generator (DC-DC)3/1 -> NOT1/1, [S_P1]
  Gain2/1 -> [Ib_ref1]
  [S_N] -> Mosfet1/1
  [S_P] -> Mosfet/1
  Constant5/1 -> Add5/1
  Voltage Measurement1/1 -> [Vload]
  [Ib_ref1] -> Add4/2
  voltage controlled1/1 -> Gain2/1
  current controlled/1 -> PWM Generator (DC-DC)3/1
  Add4/1 -> current controlled/1
  NOT1/1 -> [S_N1]
  [Vb] -> Add5/2
  [Ib] -> Add4/1
  connections:
  Series RLC Branch5/RConn1 -- charge_in-/RConn1 -- Mosfet3/RConn1 -- charge_out-/RConn1 -- Series RLC Branch6/RConn1
  Mosfet3/LConn1 -- Mosfet2/RConn1 -- Series RLC Branch4/LConn1
  Series RLC Branch5/LConn1 -- charge_in+/RConn1 -- Mosfet2/LConn1
  Series RLC Branch3/LConn1 -- disch_out+/RConn1 -- Mosfet/LConn1 -- Voltage Measurement1/LConn1
  Series RLC Branch6/LConn1 -- charge_out+/RConn1 -- Series RLC Branch7/LConn1
  Series RLC Branch3/RConn1 -- Voltage Measurement1/LConn2 -- disch_out-/RConn1 -- Mosfet1/RConn1 -- disch_in-/RConn1 -- Series RLC Branch2/RConn1
  Series RLC Branch4/RConn1 -- Series RLC Branch7/RConn1
  Mosfet/RConn1 -- Series RLC Branch1/RConn1 -- Mosfet1/LConn1
  Series RLC Branch2/LConn1 -- disch_in+/RConn1 -- Series RLC Branch1/LConn1

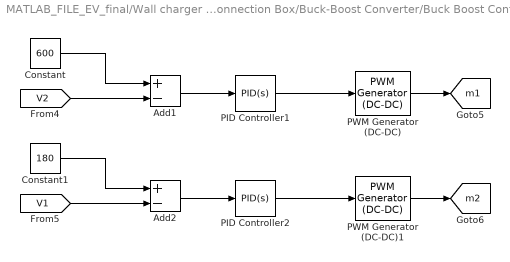
== system MATLAB_FILE_EV_final/Wall charger Connection Box/Buck-Boost Converter/Buck Boost Controller ==
  Add1 : Sum  Inputs=+-
  Add2 : Sum  Inputs=+-
  Constant : Constant  Value=600
  Constant1 : Constant  Value=180
  PID Controller1 : pid_lib/PID Controller  Controller=PID  Form=Parallel  TimeDomain=Continuous-time  UseExternalTs=off  SampleTime=-1  IntegratorMethod=Forward Euler  FilterMethod=Forward Euler  ControllerParametersSource=internal  P=0  I=7  D=0  UseFilter=on  N=100  TunerSelectOption=Transfer Function Based (PID Tuner App)  InitialConditionSource=internal  InitialConditionForIntegrator=0  InitialConditionForFilter=0  DifferentiatorICPrevScaledInput=0  ExternalReset=none  TrackingMode=off  Kt=1  LimitOutput=off  SatLimitsSource=internal  UpperSaturationLimit=inf  LowerSaturationLimit=-inf  LinearizeAsGain=on  AntiWindupMode=none  Kb=1  POutMin=[]  POutMax=[]  IOutMin=[]  IOutMax=[]  DOutMin=[]  DOutMax=[]  NOutMin=[]  NOutMax=[]  SumOutMin=[]  SumOutMax=[]  SaturationOutMin=[]  SaturationOutMax=[]  PParamMin=[]  PParamMax=[]  IParamMin=[]  IParamMax=[]  DParamMin=[]  DParamMax=[]  NParamMin=[]  NParamMax=[]  KbParamMin=[]  KbParamMax=[]  KtParamMin=[]  KtParamMax=[]  KbOutMin=[]  KbOutMax=[]  KtOutMin=[]  KtOutMax=[]  IntegratorOutMin=[]  IntegratorOutMax=[]  FilterOutMin=[]  FilterOutMax=[]  SumI1OutMin=[]  SumI1OutMax=[]  SumI2OutMin=[]  SumI2OutMax=[]  SumI3OutMin=[]  SumI3OutMax=[]  SumI4OutMin=[]  SumI4OutMax=[]  SumDOutMin=[]  SumDOutMax=[]  DifferentiatorOutMin=[]  DifferentiatorOutMax=[]  FilterDiffOutCoefMin=[]  FilterDiffOutCoefMax=[]  ReciprocalOutMin=[]  ReciprocalOutMax=[]  SumDenOutMin=[]  SumDenOutMax=[]  SumNumOutMin=[]  SumNumOutMax=[]  DivideOutMin=[]  DivideOutMax=[]  UdiffTsProdOutMin=[]  UdiffTsProdOutMax=[]  NTsProdOutMin=[]  NTsProdOutMax=[]  UintegralTsProdOutMin=[]  UintegralTsProdOutMax=[]  UngainTsProdOutMin=[]  UngainTsProdOutMax=[]  IntegratorContinuousStateAttributes=''  IntegratorStateMustResolveToSignalObject=off  IntegratorRTWStateStorageClass=Auto  FilterContinuousStateAttributes=''  FilterStateMustResolveToSignalObject=off  FilterRTWStateStorageClass=Auto  ParallelPVariant=InternalParameters  IdealPVariant=Disabled  IVariant=InternalParameters  DVariant=InternalParameters  IntegratorVariant=Continuous  SatVariant=Disabled  AWVariant=Passthrough  PCopyVariant=Disabled  TRVariant=Disabled  FdbkBlocksVariant=Forward  IdealPFdbkVariant=Disabled  SatFdbkVariant=Disabled  DerivativeFilterVariant=ContFilter  NVariant=InternalParameters  NCopyVariant=Disabled  FilterICVariant=InternalICsFilter  IntegratorICVariant=InternalICs  ExternalResetVariant=Disabled  TRSumVariant=Passthrough  SumFdbkVariant=Disabled  SumVariant=Sum_PID  TsampFilterVariant=InternalTs  TsampNgainVariant=Passthrough  TsampIntegralVariant=Passthrough  ExternalSaturationOutDataTypeStr=Inherit: Same as second input
  PID Controller2 : pid_lib/PID Controller  Controller=PID  Form=Parallel  TimeDomain=Continuous-time  UseExternalTs=off  SampleTime=-1  IntegratorMethod=Forward Euler  FilterMethod=Forward Euler  ControllerParametersSource=internal  P=0  I=7  D=0  UseFilter=on  N=100  TunerSelectOption=Transfer Function Based (PID Tuner App)  InitialConditionSource=internal  InitialConditionForIntegrator=0  InitialConditionForFilter=0  DifferentiatorICPrevScaledInput=0  ExternalReset=none  TrackingMode=off  Kt=1  LimitOutput=off  SatLimitsSource=internal  UpperSaturationLimit=inf  LowerSaturationLimit=-inf  LinearizeAsGain=on  AntiWindupMode=none  Kb=1  POutMin=[]  POutMax=[]  IOutMin=[]  IOutMax=[]  DOutMin=[]  DOutMax=[]  NOutMin=[]  NOutMax=[]  SumOutMin=[]  SumOutMax=[]  SaturationOutMin=[]  SaturationOutMax=[]  PParamMin=[]  PParamMax=[]  IParamMin=[]  IParamMax=[]  DParamMin=[]  DParamMax=[]  NParamMin=[]  NParamMax=[]  KbParamMin=[]  KbParamMax=[]  KtParamMin=[]  KtParamMax=[]  KbOutMin=[]  KbOutMax=[]  KtOutMin=[]  KtOutMax=[]  IntegratorOutMin=[]  IntegratorOutMax=[]  FilterOutMin=[]  FilterOutMax=[]  SumI1OutMin=[]  SumI1OutMax=[]  SumI2OutMin=[]  SumI2OutMax=[]  SumI3OutMin=[]  SumI3OutMax=[]  SumI4OutMin=[]  SumI4OutMax=[]  SumDOutMin=[]  SumDOutMax=[]  DifferentiatorOutMin=[]  DifferentiatorOutMax=[]  FilterDiffOutCoefMin=[]  FilterDiffOutCoefMax=[]  ReciprocalOutMin=[]  ReciprocalOutMax=[]  SumDenOutMin=[]  SumDenOutMax=[]  SumNumOutMin=[]  SumNumOutMax=[]  DivideOutMin=[]  DivideOutMax=[]  UdiffTsProdOutMin=[]  UdiffTsProdOutMax=[]  NTsProdOutMin=[]  NTsProdOutMax=[]  UintegralTsProdOutMin=[]  UintegralTsProdOutMax=[]  UngainTsProdOutMin=[]  UngainTsProdOutMax=[]  IntegratorContinuousStateAttributes=''  IntegratorStateMustResolveToSignalObject=off  IntegratorRTWStateStorageClass=Auto  FilterContinuousStateAttributes=''  FilterStateMustResolveToSignalObject=off  FilterRTWStateStorageClass=Auto  ParallelPVariant=InternalParameters  IdealPVariant=Disabled  IVariant=InternalParameters  DVariant=InternalParameters  IntegratorVariant=Continuous  SatVariant=Disabled  AWVariant=Passthrough  PCopyVariant=Disabled  TRVariant=Disabled  FdbkBlocksVariant=Forward  IdealPFdbkVariant=Disabled  SatFdbkVariant=Disabled  DerivativeFilterVariant=ContFilter  NVariant=InternalParameters  NCopyVariant=Disabled  FilterICVariant=InternalICsFilter  IntegratorICVariant=InternalICs  ExternalResetVariant=Disabled  TRSumVariant=Passthrough  SumFdbkVariant=Disabled  SumVariant=Sum_PID  TsampFilterVariant=InternalTs  TsampNgainVariant=Passthrough  TsampIntegralVariant=Passthrough  ExternalSaturationOutDataTypeStr=Inherit: Same as second input
  PWM Generator (DC-DC) : spsPWMGeneratorDCDCLib/PWM Generator (DC-DC)  Fsw=5000  Ts=0
  PWM Generator (DC-DC)1 : spsPWMGeneratorDCDCLib/PWM Generator (DC-DC)  Fsw=5000  Ts=0
  tag scope: m1=global, m2=global
  wires:
  Constant/1 -> Add1/1
  PID Controller2/1 -> PWM Generator (DC-DC)1/1
  Constant1/1 -> Add2/1
  PWM Generator (DC-DC)1/1 -> [m2]
  [V1] -> Add2/2
  PID Controller1/1 -> PWM Generator (DC-DC)/1
  PWM Generator (DC-DC)/1 -> [m1]
  Add2/1 -> PID Controller2/1
  [V2] -> Add1/2
  Add1/1 -> PID Controller1/1

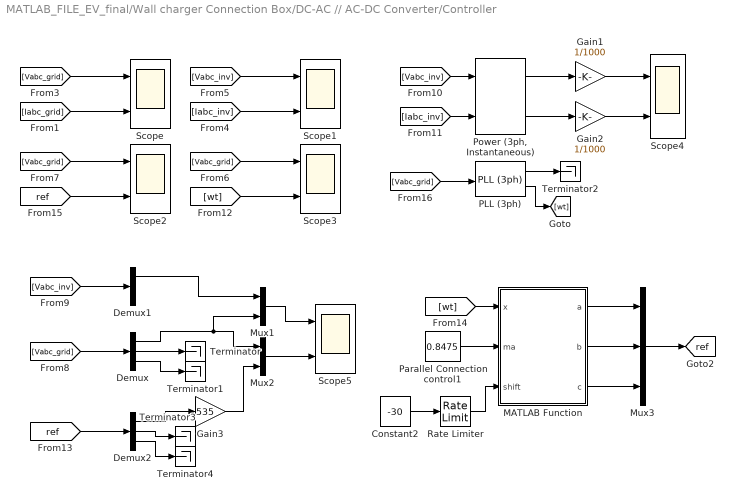
== system MATLAB_FILE_EV_final/Wall charger Connection Box/DC-AC // AC-DC Converter/Controller ==
  Constant2 : Constant  Value=-30
  Demux : Demux  Outputs=3
  Demux1 : Demux  Outputs=3
  Demux2 : Demux  Outputs=3
  Gain1 : Gain  Gain=1/1000
  Gain2 : Gain  Gain=1/1000
  Gain3 : Gain  Gain=535
  MATLAB Function : MATLAB Function  TreatAsAtomicUnit=on
  Mux1 : Mux  Inputs=2
  Mux2 : Mux  Inputs=2
  Mux3 : Mux  Inputs=3
  PLL (3ph) : spsPLL3phLib/PLL (3ph)  Fmin=45  Par_Init=[0, 50]  ParK=[180, 3200, 1]  TcD=1e-4  MaxRateChangeFreq=12  FilterCutOffFreq=25  Ts=0  AGC=on
  Parallel Connection control1 : Constant  Value=0.8475
  "Power (3ph, Instantaneous)" : spsPower3phInstantaneousLib/Power (3ph, Instantaneous)
  Rate Limiter : RateLimiter  SampleTimeMode=inherited
  Scope{,1..5} (6 alike) : Scope  NumInputPorts=2
  Terminator{,1..4} (5 alike) : Terminator
  tag scope: ref=global
  wires:
  Demux1/1 -> Mux1/1
  Mux3/1 -> [ref]
  Gain2/1 -> Scope4/2
  MATLAB Function/2(b) -> Mux3/2
  Gain3/1 -> Mux2/2
  Demux/3 -> Terminator1/1
  [ref] -> Demux2/1
  "Power (3ph, Instantaneous)"/1 -> Gain1/1
  [Iabc_inv] -> "Power (3ph, Instantaneous)"/2
  Constant2/1 -> Rate Limiter/1
  [Vabc_grid] -> PLL (3ph)/1
  Demux2/1 -> Gain3/1
  Demux/2 -> Terminator/1
  PLL (3ph)/1 -> Terminator2/1
  Parallel Connection control1/1 -> MATLAB Function/2(ma)
  "Power (3ph, Instantaneous)"/2 -> Gain2/1
  [ref] -> Scope2/2
  Gain1/1 -> Scope4/1
  [wt] -> MATLAB Function/1(x)
  [Vabc_inv] -> Scope1/1
  Demux2/2 -> Terminator3/1
  MATLAB Function/3(c) -> Mux3/3
  PLL (3ph)/2 -> [wt]
  [wt] -> Scope3/2
  Mux2/1 -> Scope5/2
  [Vabc_grid] -> Scope2/1
  [Iabc_grid] -> Scope/2
  [Iabc_inv] -> Scope1/2
  [Vabc_inv] -> Demux1/1
  Rate Limiter/1 -> MATLAB Function/3(shift)
  Mux1/1 -> Scope5/1
  [Vabc_grid] -> Scope3/1
  [Vabc_inv] -> "Power (3ph, Instantaneous)"/1
  Demux2/3 -> Terminator4/1
  Demux/1 -> Mux1/2, Mux2/1
  [Vabc_grid] -> Scope/1
  MATLAB Function/1(a) -> Mux3/1
  [Vabc_grid] -> Demux/1
